simulink model "G1"  (R2015a)
settings: Solver=ode3  StartTime=0.0  StopTime=15  FixedStep=0.01  RelTol=1e-3
InitFcn:
  | Ku = 4.6737;
  | Tu = 3.26;
  | Kpmin = 0.32*Ku;
  | Kpmax = 0.6*Ku;
  | Kdmin = 0.08*Ku*Tu;
  | Kdmax = 0.15*Ku*Tu;
libraries: simulink x2, fuzblock x1
settings Model: Creator=sahandar  LastModifiedBy=sahandar

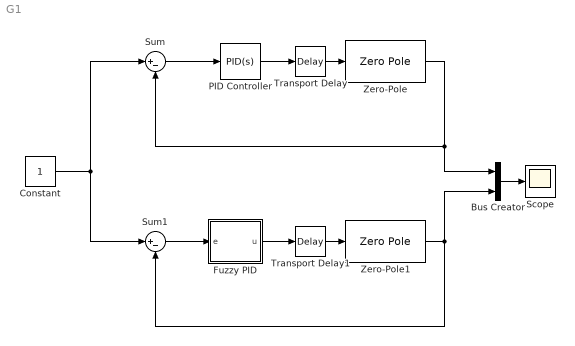
== system G1 ==
  Bus Creator : BusCreator  Inputs=2
  Constant : Constant
  Fuzzy PID : Subsystem
  PID Controller : simulink/Continuous/PID Controller  Controller=PID  TimeDomain=Continuous-time  SampleTime=-1  IntegratorMethod=Forward Euler  FilterMethod=Forward Euler  Form=Parallel  UseFilter=on  ControllerParametersSource=internal  P=0.6*Ku  I=1.2*Ku/Tu  D=0.6*Ku*Tu/8  N=100  InitialConditionSource=internal  InitialConditionForIntegrator=0  InitialConditionForFilter=0  ExternalReset=none  LimitOutput=off  UpperSaturationLimit=inf  LowerSaturationLimit=-inf  LinearizeAsGain=on  AntiWindupMode=none  Kb=1  TrackingMode=off  Kt=1  PParamMin=[]  PParamMax=[]  IParamMin=[]  IParamMax=[]  DParamMin=[]  DParamMax=[]  NParamMin=[]  NParamMax=[]  KbParamMin=[]  KbParamMax=[]  KtParamMin=[]  KtParamMax=[]  POutMin=[]  POutMax=[]  IOutMin=[]  IOutMax=[]  DOutMin=[]  DOutMax=[]  NOutMin=[]  NOutMax=[]  KbOutMin=[]  KbOutMax=[]  KtOutMin=[]  KtOutMax=[]  IntegratorOutMin=[]  IntegratorOutMax=[]  FilterOutMin=[]  FilterOutMax=[]  SumOutMin=[]  SumOutMax=[]  SumI1OutMin=[]  SumI1OutMax=[]  SumI2OutMin=[]  SumI2OutMax=[]  SumI3OutMin=[]  SumI3OutMax=[]  SumDOutMin=[]  SumDOutMax=[]  SaturationOutMin=[]  SaturationOutMax=[]  IntegratorContinuousStateAttributes=''  IntegratorStateMustResolveToSignalObject=off  IntegratorRTWStateStorageClass=Auto  FilterContinuousStateAttributes=''  FilterStateMustResolveToSignalObject=off  FilterRTWStateStorageClass=Auto  DifferentiatorICPrevScaledInput=0  DifferentiatorOutMin=[]  DifferentiatorOutMax=[]
  Scope : Scope
      settings: YMin=0.00525  YMax=0.009
  Sum : Sum  Inputs=|+-
  Sum1 : Sum  Inputs=|+-
  Transport Delay : TransportDelay  DelayTime=0.5
  Transport Delay1 : TransportDelay  DelayTime=0.5
  Zero-Pole : ZeroPole  Zeros=[]  Poles=[-1 -1]  Gain=1
  Zero-Pole1 : ZeroPole  Zeros=[]  Poles=[-1 -1]  Gain=1
  wires:
  Transport Delay/1 -> Zero-Pole/1
  PID Controller/1 -> Transport Delay/1
  Sum/1 -> PID Controller/1
  Constant/1 -> Sum/1, Sum1/1
  Zero-Pole/1 -> Sum/2, Bus Creator/1
  Transport Delay1/1 -> Zero-Pole1/1
  Zero-Pole1/1 -> Sum1/2, Bus Creator/2
  Bus Creator/1 -> Scope/1
  Sum1/1 -> Fuzzy PID/1(e)
  Fuzzy PID/1(u) -> Transport Delay1/1

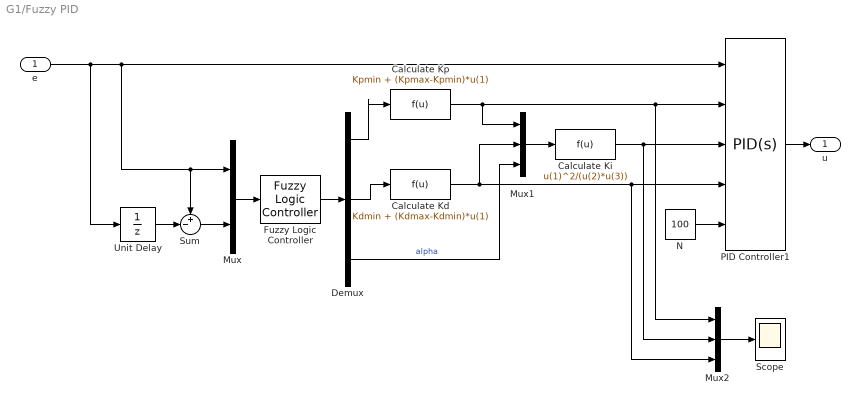
== system G1/Fuzzy PID ==
  e : Inport
  Calculate Kd : Fcn  Expr=Kdmin + (Kdmax-Kdmin)*u(1)
  Calculate Ki : Fcn  Expr=u(1)^2/(u(2)*u(3))
  Calculate Kp : Fcn  Expr=Kpmin + (Kpmax-Kpmin)*u(1)
  Demux : Demux  Outputs=3
  Fuzzy Logic Controller : fuzblock/Fuzzy Logic  Controller  fis='fuzzy_pid.fis'
  Mux : Mux  Inputs=2
  Mux1 : Mux  Inputs=3
  Mux2 : Mux  Inputs=3
  N : Constant  Value=100
  PID Controller1 : simulink/Continuous/PID Controller  Controller=PID  TimeDomain=Continuous-time  SampleTime=-1  IntegratorMethod=Forward Euler  FilterMethod=Forward Euler  Form=Parallel  UseFilter=on  ControllerParametersSource=external  P=0.6*4.6737  I=1.2*4.6737/3.26  D=0.6*4.6737*3.26/8  N=100  InitialConditionSource=internal  InitialConditionForIntegrator=0  InitialConditionForFilter=0  ExternalReset=none  LimitOutput=off  UpperSaturationLimit=inf  LowerSaturationLimit=-inf  LinearizeAsGain=on  AntiWindupMode=none  Kb=1  TrackingMode=off  Kt=1  PParamMin=[]  PParamMax=[]  IParamMin=[]  IParamMax=[]  DParamMin=[]  DParamMax=[]  NParamMin=[]  NParamMax=[]  KbParamMin=[]  KbParamMax=[]  KtParamMin=[]  KtParamMax=[]  POutMin=[]  POutMax=[]  IOutMin=[]  IOutMax=[]  DOutMin=[]  DOutMax=[]  NOutMin=[]  NOutMax=[]  KbOutMin=[]  KbOutMax=[]  KtOutMin=[]  KtOutMax=[]  IntegratorOutMin=[]  IntegratorOutMax=[]  FilterOutMin=[]  FilterOutMax=[]  SumOutMin=[]  SumOutMax=[]  SumI1OutMin=[]  SumI1OutMax=[]  SumI2OutMin=[]  SumI2OutMax=[]  SumI3OutMin=[]  SumI3OutMax=[]  SumDOutMin=[]  SumDOutMax=[]  SaturationOutMin=[]  SaturationOutMax=[]  IntegratorContinuousStateAttributes=''  IntegratorStateMustResolveToSignalObject=off  IntegratorRTWStateStorageClass=Auto  FilterContinuousStateAttributes=''  FilterStateMustResolveToSignalObject=off  FilterRTWStateStorageClass=Auto  DifferentiatorICPrevScaledInput=0  DifferentiatorOutMin=[]  DifferentiatorOutMax=[]
  Scope : Scope
  Sum : Sum  Inputs=+-|
  Unit Delay : UnitDelay  SampleTime=-1
  u : Outport
  wires:
  PID Controller1/1 -> u/1
  e/1 -> Unit Delay/1, PID Controller1/1, Sum/1, Mux/1
  N/1 -> PID Controller1/5
  Mux/1 -> Fuzzy Logic Controller/1
  Fuzzy Logic Controller/1 -> Demux/1
  Demux/1 -> Calculate Kp/1
  Calculate Kp/1 -> Mux2/1, PID Controller1/2, Mux1/1
  Demux/2 -> Calculate Kd/1
  Calculate Kd/1 -> Mux1/2, Mux2/3, PID Controller1/4
  Calculate Ki/1 -> Mux2/2, PID Controller1/3
  Mux1/1 -> Calculate Ki/1
  Demux/3 -> Mux1/3  "alpha"
  Sum/1 -> Mux/2
  Unit Delay/1 -> Sum/2
  Mux2/1 -> Scope/1
